simulink model "pendulodaniel"  (R2013a)
settings: Solver=ode45  StartTime=0.0  StopTime=300  RelTol=1e-3
values from neighbouring files (symbols this model uses):
  R = 1.08985886328    [R.mat]    (also in S.mat)
  S = 8.175    [R.mat]    (also in S.mat)
undefined symbols (not defined in the file or in its folder): bace, pendulo, pendulodaniel, RootGround, RootPart
libraries: mblibv1 x9
settings Model: Creator=Daniel  LastModifiedBy=Daniel
settings SimMechanicsCC: VisOnUpdateDiagram=on  VisDuringSimulation=on

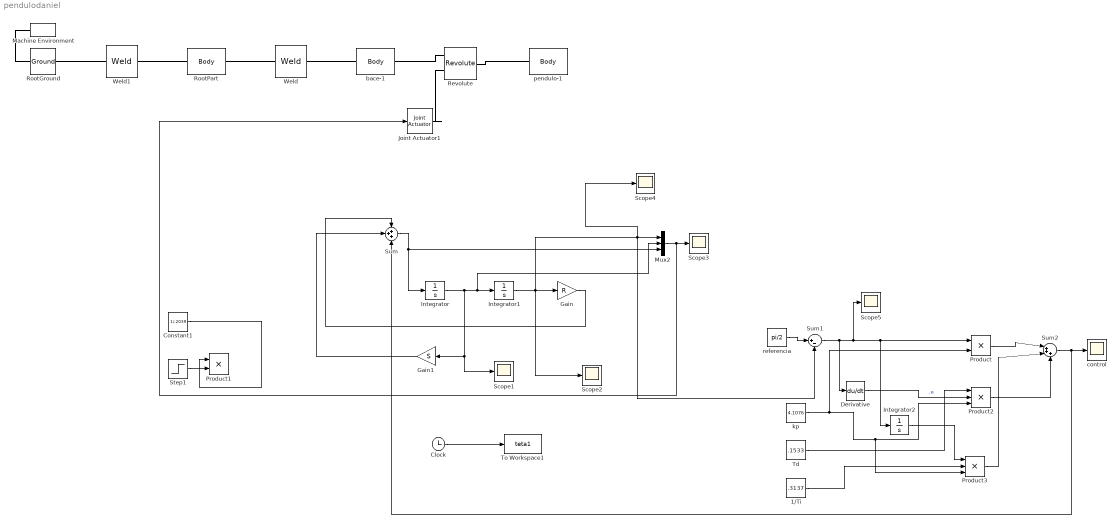
== system pendulodaniel ==
  1/Ti : Constant  Value=.3137
  Clock : Clock
  Constant1 : Constant  Value=1/.2039
  Derivative : Derivative
  Gain : Gain  Gain=R
  Gain1 : Gain  Gain=S
  Integrator : Integrator
  Integrator1 : Integrator
  Integrator2 : Integrator
  Joint Actuator1 : mblibv1/Sensors &  Actuators/Joint Actuator  UpdateFromCAD=off  PhysicalDomain=Mechanical  PortType=blob  ActuationStyle=Motion  AngleUnits=rad  ArcVelocityUnits=rad/s  ArcAccelerationUnits=rad/s^2  CoordPositionUnits=m  VelocityUnits=m/s  AccelerationUnits=m/s^2  ForceUnits=mN  TorqueUnits=N*m  ActiveIO=on  Width=3  DialogClass=MechanicalActuatorBlock  Primitive=R1  ReferenceFrame=Absolute (World)
  Machine Environment : mblibv1/Bodies/Machine Environment  PortType=env  PhysicalDomain=Mechanical  DialogTemplateClass=MECH.MachineEnvironment  SyncWhenCopied=off  Gravity=[0 -9.81 0]  GravityUnits=m/s^2  GravityAsSignal=off  Dimensionality=Auto-detect  AnalysisType=Forward dynamics  LinearAssemblyTolerance=1e-3  LinearAssemblyToleranceUnits=m  AngularAssemblyTolerance=1e-3  AngularAssemblyToleranceUnits=rad  ConstraintSolverType=Stabilizing  ConstraintRelTolerance=1e-4  ConstraintAbsTolerance=1e-4  UseRobustSingularityHandling=off  RedundancyAnalysisToleranceType=Automatically select tolerance  RedundancyAnalysisTolerance=1e-14  StatePerturbationType=Fixed  PerturbationSize=1e-5  VisualizeMachine=on  BodyVisualizationType=Use model default body geometries  BodyColorSelMode=Use model default  DefaultBodyColor=[1 0 0]
  Mux2 : Mux  Inputs=3
  Product : Product
  Product1 : Product
  Product2 : Product  Inputs=3
  Product3 : Product  Inputs=3
  Revolute : mblibv1/Joints/Revolute  LConnTagsString=__newl0|SA1  RConnTagsString=__newr0  UpdateFromCAD=on  PMImportedID=bace-1:-:pendulo-1  NumSAPorts=1  CutJoint=off  MarkAsCut=off  Primitives=prismatic  PrimitiveProps=R1$World$[0,0,1]$revolute  DialogClass=JointBlock  R1Axis=[0,0,1]
  RootGround : mblibv1/Bodies/Ground  UpdateFromCAD=on  PMImportedID=RootGround  LeftPortType=env  RightPortType=workingframe  PhysicalDomain=Mechanical  DialogClass=GroundBlock  CoordPosition=[-0.280972,0.108441,0.646305]  CoordPositionUnits=m  StateVectorMgrId=1  MachineId=[2 0]  ShowEnvPort=on
  RootPart : mblibv1/Bodies/Body  LConnTagsString=CS3  RConnTagsString=CS2  UpdateFromCAD=on  PMImportedID=pendulodaniel/RootPart  DialogClass=MechanicalBodyBlock  Mass=0  MassUnits=kg  InertiaUnits=kg*m^2  Inertia=[0,0,0;0,0,0;0,0,0]  Shape=Cylinder  ShapeDims=[1 1]  ShapeUnits=m  ShapeUse=false  Density=1  DensityUnits=kg/m^3  DensityUse=false  GraphicsMode=MACHINE_DEFAULT  BodyColorSelMode=MACHINE_DEFAULT  BodyColor=[1;0;0]  AttachedToCS=CS1  CG=Right$CG$[-0.280972 0.108441 0.646305]$WORLD$WORLD$m$[1 0 0;0 1 0;0 0 1]$3x3 Transform$rad$WORLD$false$pendulodaniel/RootPart::CG(AUTOGEN)  WorkingFrames=Right$CS1$[0 0 0]$WORLD$WORLD$m$[1 0 0;0 1 0;0 0 1]$3x3 Transform$rad$WORLD$false$pendulodaniel/RootPart::CS1(AUTOGEN)#Right$CS2$[-0.332044 0.120792 0.65]$WORLD$WORLD$m$[1 0 0;0 1 0;0 0 1]$3x3 Transform$rad$WORLD$true$bace-1:-:pendulodaniel/RootPart::pendulodaniel/RootPart(AUTOGEN)#Left$CS3$[-0.280972 0.108441 0.646305]$WORLD$WORLD$m$[1 0 0;0 1 0;0 0 1]$3x3 Transform$rad$WORLD$true$RootGround:-:pendulodaniel/RootPart::pendulodaniel/RootPart(AUTOGEN)  CGPos=[-0.280972 0.108441 0.646305]  CGRot=[1 0 0;0 1 0;0 0 1]  CS0Pos=[]  CS0Rot=[]  CS1Pos=[0 0 0]  CS1Rot=[1 0 0;0 1 0;0 0 1]  CS2Pos=[-0.332044 0.120792 0.65]  CS2Rot=[1 0 0;0 1 0;0 0 1]  CS3Pos=[-0.280972 0.108441 0.646305]  CS3Rot=[1 0 0;0 1 0;0 0 1]  CS4Pos=[]  CS4Rot=[]  CS5Pos=[]  CS5Rot=[]  CS6Pos=[]  CS6Rot=[]  CS7Pos=[]  CS7Rot=[]  CS8Pos=[]  CS8Rot=[]  CS9Pos=[]  CS9Rot=[]  CS10Pos=[]  CS10Rot=[]  CS11Pos=[]  CS11Rot=[]  CS12Pos=[]  CS12Rot=[]  CS13Pos=[]  CS13Rot=[]  CS14Pos=[]  CS14Rot=[]  CS15Pos=[]  CS15Rot=[]  CS16Pos=[]  CS16Rot=[]  CS17Pos=[]  CS17Rot=[]  CS18Pos=[]  CS18Rot=[]  CS19Pos=[]  CS19Rot=[]  CS20Pos=[]  CS20Rot=[]
  Scope{1..5} (5 alike) : Scope
      Scope1 settings: YMin=0.033158  YMax=0.0366484  SaveName=ScopeData2
      Scope2 settings: YMin=0.3  YMax=0.3004  SaveName=ScopeData4
      Scope3 settings: YMin=0.033158  YMax=0.0366484  SaveName=ScopeData3
      Scope4 settings: YMin=0.299965  YMax=0.300005  SaveName=wero
      Scope5 settings: YMin=0.299965  YMax=0.300005  SaveName=wero1
  Step1 : Step  Time=3  SampleTime=0
  Sum : Sum  Inputs=+++
  Sum1 : Sum  Inputs=|+-
  Sum2 : Sum  Inputs=|+++
  Td : Constant  Value=.1533
  To Workspace1 : ToWorkspace  VariableName=teta1  SampleTime=-1
  Weld : mblibv1/Joints/Weld  LConnTagsString=__newl0  RConnTagsString=__newr0  UpdateFromCAD=on  PMImportedID=bace-1:-:pendulodaniel/RootPart  NumSAPorts=0  CutJoint=off  MarkAsCut=off  Primitives=weld  PrimitiveProps=W$WORLD$[0.57735,0.57735,0.57735]$weld  DialogClass=JointBlock  WAxis=[0.57735,0.57735,0.57735]
  Weld1 : mblibv1/Joints/Weld  LConnTagsString=__newl0  RConnTagsString=__newr0  UpdateFromCAD=on  PMImportedID=RootGround:-:pendulodaniel/RootPart  NumSAPorts=0  CutJoint=off  MarkAsCut=off  Primitives=weld  PrimitiveProps=W$WORLD$[0.57735,0.57735,0.57735]$weld  DialogClass=JointBlock  WAxis=[0.57735,0.57735,0.57735]
  bace-1 : mblibv1/Bodies/Body  LConnTagsString=CS2  RConnTagsString=CS3  UpdateFromCAD=on  PMImportedID=bace-1  DialogClass=MechanicalBodyBlock  Mass=27.0254  MassUnits=kg  InertiaUnits=kg*m^2  Inertia=[0.861562,-0.538434,0;-0.538434,1.01646,0;0,0,1.87397]  Shape=Cylinder  ShapeDims=[1 1]  ShapeUnits=m  ShapeUse=false  Density=1  DensityUnits=kg/m^3  DensityUse=false  GraphicsMode=GFXFILE  GraphicsFileName=pendulodaniel - bace-1.STL  BodyColorSelMode=COLORPALETTE  BodyColor=[1;1;0]  AttachedToCS=CS1  CG=Right$CG$[-0.332044 0.120792 0.65]$WORLD$WORLD$m$[1 0 0;0 1 0;0 0 1]$3x3 Transform$rad$WORLD$false$bace-1::CG(AUTOGEN)  WorkingFrames=Right$CS1$[-0.533119 -0.297332 0.635]$WORLD$WORLD$m$[1 0 0;0 1 0;0 0 1]$3x3 Transform$rad$WORLD$false$bace-1::CS1(AUTOGEN)#Left$CS2$[-0.332044 0.120792 0.65]$WORLD$WORLD$m$[1 0 0;0 1 0;0 0 1]$3x3 Transform$rad$WORLD$true$bace-1:-:pendulodaniel/RootPart::bace-1(AUTOGEN)#Right$CS3$[0.0668806 0.252668 0.665]$WORLD$WORLD$m$[1 0 0;0 1 0;0 0 1]$3x3 Transform$rad$WORLD$true$bace-1:-:pendulo-1::bace-1(AUTOGEN)  CGPos=[-0.332044 0.120792 0.65]  CGRot=[1 0 0;0 1 0;0 0 1]  CS0Pos=[]  CS0Rot=[]  CS1Pos=[-0.533119 -0.297332 0.635]  CS1Rot=[1 0 0;0 1 0;0 0 1]  CS2Pos=[-0.332044 0.120792 0.65]  CS2Rot=[1 0 0;0 1 0;0 0 1]  CS3Pos=[0.0668806 0.252668 0.665]  CS3Rot=[1 0 0;0 1 0;0 0 1]  CS4Pos=[]  CS4Rot=[]  CS5Pos=[]  CS5Rot=[]  CS6Pos=[]  CS6Rot=[]  CS7Pos=[]  CS7Rot=[]  CS8Pos=[]  CS8Rot=[]  CS9Pos=[]  CS9Rot=[]  CS10Pos=[]  CS10Rot=[]  CS11Pos=[]  CS11Rot=[]  CS12Pos=[]  CS12Rot=[]  CS13Pos=[]  CS13Rot=[]  CS14Pos=[]  CS14Rot=[]  CS15Pos=[]  CS15Rot=[]  CS16Pos=[]  CS16Rot=[]  CS17Pos=[]  CS17Rot=[]  CS18Pos=[]  CS18Rot=[]  CS19Pos=[]  CS19Rot=[]  CS20Pos=[]  CS20Rot=[]
  control : Scope
      settings: YMin=77.5  YMax=84
  kp : Constant  Value=4.1076
  pendulo-1 : mblibv1/Bodies/Body  LConnTagsString=CS2  UpdateFromCAD=on  PMImportedID=pendulo-1  DialogClass=MechanicalBodyBlock  Mass=4.10166  MassUnits=kg  InertiaUnits=kg*m^2  Inertia=[0.0742579,0,0;0,0.0762547,0.00181393;0,0.00181393,0.00306232]  Shape=Cylinder  ShapeDims=[1 1]  ShapeUnits=m  ShapeUse=false  Density=1  DensityUnits=kg/m^3  DensityUse=false  GraphicsMode=GFXFILE  GraphicsFileName=pendulodaniel - pendulo-1.STL  BodyColorSelMode=COLORPALETTE  BodyColor=[0.478431;0.0627451;0.894118]  AttachedToCS=CS1  CG=Right$CG$[0.0555329 0.0270573 0.621958]$WORLD$WORLD$m$[0.998737 0 -0.0502339;-0.0502339 0 -0.998737;0 1 0]$3x3 Transform$rad$WORLD$false$pendulo-1::CG(AUTOGEN)  WorkingFrames=Right$CS1$[0.0325595 -0.131092 0.605]$WORLD$WORLD$m$[0.998737 0 -0.0502339;-0.0502339 0 -0.998737;0 1 0]$3x3 Transform$rad$WORLD$false$pendulo-1::CS1(AUTOGEN)#Left$CS2$[0.0668806 0.252668 0.665]$WORLD$WORLD$m$[1 0 0;0 1 0;0 0 1]$3x3 Transform$rad$WORLD$true$bace-1:-:pendulo-1::pendulo-1(AUTOGEN)  CGPos=[0.0555329 0.0270573 0.621958]  CGRot=[0.998737 0 -0.0502339;-0.0502339 0 -0.998737;0 1 0]  CS0Pos=[]  CS0Rot=[]  CS1Pos=[0.0325595 -0.131092 0.605]  CS1Rot=[0.998737 0 -0.0502339;-0.0502339 0 -0.998737;0 1 0]  CS2Pos=[0.0668806 0.252668 0.665]  CS2Rot=[1 0 0;0 1 0;0 0 1]  CS3Pos=[]  CS3Rot=[]  CS4Pos=[]  CS4Rot=[]  CS5Pos=[]  CS5Rot=[]  CS6Pos=[]  CS6Rot=[]  CS7Pos=[]  CS7Rot=[]  CS8Pos=[]  CS8Rot=[]  CS9Pos=[]  CS9Rot=[]  CS10Pos=[]  CS10Rot=[]  CS11Pos=[]  CS11Rot=[]  CS12Pos=[]  CS12Rot=[]  CS13Pos=[]  CS13Rot=[]  CS14Pos=[]  CS14Rot=[]  CS15Pos=[]  CS15Rot=[]  CS16Pos=[]  CS16Rot=[]  CS17Pos=[]  CS17Rot=[]  CS18Pos=[]  CS18Rot=[]  CS19Pos=[]  CS19Rot=[]  CS20Pos=[]  CS20Rot=[]
  referencia : Constant  Value=pi/2
  wires:
  Integrator/1 -> Scope1/1, Gain1/1, Mux2/2, Integrator1/1
  Clock/1 -> To Workspace1/1
  Sum/1 -> Integrator/1, Mux2/3
  Constant1/1 -> Product1/1
  Step1/1 -> Product1/2
  Mux2/1 -> Joint Actuator1/1, Scope3/1
  referencia/1 -> Sum1/1
  Sum1/1 -> Derivative/1, Scope5/1, Product/1, Integrator2/1
  kp/1 -> Product/2, Product3/3, Product2/3
  Product/1 -> Sum2/1
  Gain/1 -> Sum/1
  1/Ti/1 -> Product3/2
  Product2/1 -> Sum2/3
  Sum2/1 -> Sum/3, control/1
  Derivative/1 -> Product2/2  ".e"
  Td/1 -> Product2/1
  Product3/1 -> Sum2/2
  Integrator2/1 -> Product3/1
  Integrator1/1 -> Scope2/1, Gain/1, Sum1/2, Scope4/1, Mux2/1
  Gain1/1 -> Sum/2
  connections:
  RootPart/RConn1 -- Weld/LConn1
  Weld/RConn1 -- bace-1/LConn1
  bace-1/RConn1 -- Revolute/LConn1
  Revolute/RConn1 -- pendulo-1/LConn1
  RootGround/RConn1 -- Weld1/LConn1
  Weld1/RConn1 -- RootPart/LConn1
  RootGround/LConn1 -- Machine Environment/RConn1
  Joint Actuator1/RConn1 -- Revolute/LConn2
